simulink model "rev0BB"  (R2017b)
settings: Solver=FixedStepDiscrete  StartTime=0  StopTime=(((preLen+100+dataLenSymbols)*1+pad_first*3)*basePer)  RelTol=1e-3
values from neighbouring files (symbols this model uses):
  ack_stf_len_symbols = length(x_ACK_STF)    [rev0BB_setup.m]
  agc_delay_lag = 32    [rev0BB_setup.m]
  agc_detector_coef = ones(1,agc_detector_taps)./agc_detector_taps    [rev0BB_setup.m]
  agc_on = true    [rev0BB_startup.m]
  agc_sat_low = -agcSaturation    (= -12)    [rev0BB_setup.m]
  agc_sat_up = agcSaturation    (= 12)    [rev0BB_setup.m]
  agcDesired = 0    [rev0BB_setup.m]
  agcExpDomain = agcSaturation    (= 12)    [rev0BB_setup.m]
  agcExpResolution = 2^-5    (= 0.03125)    [rev0BB_setup.m]
  agcPwrAvgNum = 128    [rev0BB_setup.m]
  agcSaturation = 12    [rev0BB_setup.m]
  agcSettleThresh = 0.65    [rev0BB_setup.m]
  agcStep = 2^-8    (= 0.00390625)    [rev0BB_setup.m]
  atanDomain = 5    [rev0BB_setup.m]
  atanDomainTiming = 256    [rev0BB_setup.m]
  atanResolution = 2^-9    (= 0.001953125)    [rev0BB_setup.m]
  atanResolutionTiming = 2^-5    (= 0.03125)    [rev0BB_setup.m]
  averaging_num = ones(1, averaging_samples)    [rev0BB_setup.m]
  averaging_samples = 128    [rev0BB_setup.m]
  awgnSeed = abs(dBSnrRange(dBSnrInd)*1000+trial+10000000)    [plotBer.m]    (also in rev0BB_startup.m = 67)
  basePer = 1/baseFreq    (= 5e-08)    [rev0BB_setup.m]
  bitsPerSymbolHeader = log2(radixHeader)    [rev0BB_setup.m]
  bitsPerSymbolMax = log2(radixMax)    [rev0BB_setup.m]
  cal_sig_i_mult = 1.0    (= 1)    [rev0BB_startup.m]
  cal_sig_i_offset = 0.0    (= 0)    [rev0BB_startup.m]
  cal_sig_q_mult = 1.0    (= 1)    [rev0BB_startup.m]
  cal_sig_q_offset = 0.0    (= 0)    [rev0BB_startup.m]
  cefEarlyWarning = 256    [rev0BB_setup.m]
  cefLen = length(x_CEF)    [rev0BB_setup.m]
  channelFIR = zeros(1, round(maxSampleDelay)+1)    [rev0BB_startup.m]
  coarseCFOAdaptDelay = 1    [rev0BB_setup.m]
  cr_i = 0.020    (= 0.02)    [rev0BB_setup.m]
  cr_i_preamp = 2^-9    (= 0.001953125)    [rev0BB_setup.m]
  cr_int1_sat_low = -cr_integrator1_saturation    (= -0.6)    [rev0BB_setup.m]
  cr_int1_sat_up = cr_integrator1_saturation    (= 0.6)    [rev0BB_setup.m]
  cr_integrator1_decay = 1    [rev0BB_setup.m]
  cr_integrator1_saturation = 0.6    [rev0BB_setup.m]
  cr_mult_pipeline = 0    [rev0BB_setup.m]
  cr_p = 0.015    [rev0BB_setup.m]
  cr_sat2_low = -cr_saturation2    (= -0.6)    [rev0BB_setup.m]
  cr_sat2_up = cr_saturation2    (= 0.6)    [rev0BB_setup.m]
  cr_smooth_num = (1/cr_smooth_samples).*ones(1, cr_smooth_samples)    [rev0BB_setup.m]
  D_128 = [ 1,  8,  2,  4, 16, 32, 64]    [golay.m]    (also in rev0BB_setup.m)
  D_32 = [ 1,  4,  8,  2, 16]    [golay.m]    (also in rev0BB_setup.m)
  dataLenSymbols = header_len_bytes*8/bitsPerSymbolHeader + frame_len_bytes*8/bitsPerSymbol    [rev0BB_setup.m]
  default_channel = 3    [rev0BB_setup.m]
  dmm_coefs = ones(1,dmm_samples)./dmm_samples    [rev0BB_setup.m]
  dst_field_len = 8    [rev0BB_setup.m]
  expDomain = 3.3    [rev0BB_setup.m]
  expResolution = 2^-5    (= 0.03125)    [rev0BB_setup.m]
  expTol = .1    (= 0.1)    [rev0BB_setup.m]
  flush_delay = regular_pipeline*2+mult_pipeline+4    (= 4)    [rev0BB_setup.m]
  frac_lut_domain = 256    [rev0BB_setup.m]
  frac_lut_domain_cr = 64    [rev0BB_setup.m]
  frac_lut_range_max = 512    [rev0BB_setup.m]
  frac_lut_range_max_coarse_cfo = 127    [rev0BB_setup.m]
  frac_lut_range_max_cr = 127    [rev0BB_setup.m]
  frac_lut_range_min = -frac_lut_range_max    (= -512)    [rev0BB_setup.m]
  frac_lut_range_min_coarse_cfo = -frac_lut_range_max_coarse_cfo    (= -127)    [rev0BB_setup.m]
  frac_lut_range_min_cr = -frac_lut_range_max_cr    (= -127)    [rev0BB_setup.m]
  frac_lut_table_breaks = -frac_lut_domain:frac_lut_res:(frac_lut_domain-1)    [rev0BB_setup.m]
  frac_lut_table_breaks_coarse_cfo = -frac_lut_domain_coarse_cfo:frac_lut_res_coarse_cfo:(frac_lut_domain_coarse_cfo-1)    [rev0BB_setup.m]
  frac_lut_table_breaks_cr = -frac_lut_domain_cr:frac_lut_res_cr:(frac_lut_domain_cr-1)    [rev0BB_setup.m]
  frac_lut_table_data = 1./frac_lut_table_breaks    [rev0BB_setup.m]
  frac_lut_table_data_coarse_cfo = 1./frac_lut_table_breaks_coarse_cfo    [rev0BB_setup.m]
  frac_lut_table_data_cr = 1./frac_lut_table_breaks_cr    [rev0BB_setup.m]
  freeze_en_agc = true    [rev0BB_startup.m]
  freeze_en_cr_int1 = false    [rev0BB_startup.m]
  freeze_en_cr_int2 = false    [rev0BB_startup.m]
  freeze_en_cr_phase = false    [rev0BB_startup.m]
  freeze_en_tr_int1 = false    [rev0BB_startup.m]
  freeze_en_tr_int2 = false    [rev0BB_startup.m]
  freeze_en_tr_phase = false    [rev0BB_startup.m]
  freeze_on_cef_done = true    [rev0BB_startup.m]
  freeze_on_stf_done = false    [rev0BB_startup.m]
  freeze_on_valid = true    [rev0BB_startup.m]
  golay_type = 32    [rev0BB_setup.m]
  guardInt = int16(4)    [rev0BB_setup.m]
  guardTol = int16(5)    [rev0BB_setup.m]
  header_len_bytes = 8    [rev0BB_setup.m]
  lineWidth = 60    [rev0BB_setup.m]
  lmsEqDepth = 38    [rev0BB_setup.m]
  lmsStep_init = 0.006    [rev0BB_setup.m]
  lmsStep_meta = (lmsStep_final - lmsStep_init)/cefLen    [rev0BB_setup.m]
  lnDomain = 16    [rev0BB_setup.m]
  lnResolution = 2^-5    (= 0.03125)    [rev0BB_setup.m]
  local_node_id = 2    [rev0BB_startup.m]
  maxMsgSize = length(xSpectrum_PRE)+dataLenSymbols+300    [rev0BB_setup.m]
  minSTFPeaks = 3    [rev0BB_setup.m]
  mod_scheme_len_bytes = 1    [rev0BB_setup.m]
  modBPS = [1, 2, 4]    [rev0BB_setup.m]
  modKeys = [0, 1, 2]    [rev0BB_setup.m]
  mult_pipeline = 0    [rev0BB_setup.m]
  overSampleFreq = 80e6    (= 80000000)    [rev0BB_setup.m]
  overSamplePer = 1/overSampleFreq    (= 1.25e-08)    [rev0BB_setup.m]
  pad_first = 1000    [createTestVectors.m]
  post_cr_i_offset = 0    [rev0BB_startup.m]
  post_cr_q_offset = 0    [rev0BB_startup.m]
  preambleSequentialDetect = 2    [rev0BB_setup.m]
  preLen = length(x_PRE)    [rev0BB_setup.m]
  qam16_demod_scale_factor = qam16_hdl_distance/qam16_power_normalized_distance    [rev0BB_setup.m]
  rcRxFilt = [0.000303163120401141 -0.00118915940834234 -0.00187387637177 -0.00124167532697737 0.00029186889076529 0.00164526160586517 0.00182432050803312 0.000652133621739543 -0.00105668254004908 -0.00204011570659167 -0.00150058088768918 0.00026138356356816 0.0019831869994874 0.00231075800085521 0.000821993419120097 -0.00154687337975486 -0.00305430783933469 -0.00238186490079127 0.000301216962040692 0.00325307 ...(+2001 chars)    [rev0BB_setup.m]
  rcTxFilt = [0.000303163120401141 -0.00118915940834234 -0.00187387637177 -0.00124167532697737 0.00029186889076529 0.00164526160586517 0.00182432050803312 0.000652133621739543 -0.00105668254004908 -0.00204011570659167 -0.00150058088768918 0.00026138356356816 0.0019831869994874 0.00231075800085521 0.000821993419120097 -0.00154687337975486 -0.00305430783933469 -0.00238186490079127 0.000301216962040692 0.00325307 ...(+2001 chars)    [rev0BB_setup.m]
  regular_pipeline = 0    [rev0BB_setup.m]
  rx_gain = 1    [rev0BB_setup.m]
  rx_gain_i = 1    [rev0BB_setup.m]
  rx_gain_q = 1    [rev0BB_setup.m]
  rx_impare_i_offset = 0    [rev0BB_startup.m]
  rx_impare_i_scale = 1    [rev0BB_startup.m]
  rx_impare_q_offset = 0    [rev0BB_startup.m]
  rx_impare_q_scale = 1    [rev0BB_startup.m]
  rx_offset_correction_i = 0    [rev0BB_startup.m]
  rx_offset_correction_q = 0    [rev0BB_startup.m]
  sin_source_amp = 1    [rev0BB_setup.m]
  sin_source_freq = 250e6/16    (= 15625000)    [rev0BB_setup.m]
  slowPer = overSamplePer*slowSample    (= 2.5e-08)    [rev0BB_setup.m]
  std_pkt_type = 0    [rev0BB_setup.m]
  stfLen = length(x_STF)    [rev0BB_setup.m]
  testMsg = cat(1, xCTRL_PRE_adj, header, payload)    [plotBer.m]
  timing_i = 0.25    [rev0BB_setup.m]
  ... (+25 more)
undefined symbols (not defined in the file or in its folder): cr_integrator2_saturation, doppler, i, magnitude, useFadingChannel
libraries: helperLib x128, simulink x90, golayLib x34, dspsigops x32, commfilt2 x27, commdigbbndpm3 x8, hdlsllib x6, dsparch4 x4, commdigbbndam3 x4, commchan3 x2, commrflib2 x2, commcrc2 x2
(part 8 of 10)

== system rev0BB/receiver/slow_rx_baseband_outer/slow_rx_baseband_enabled/slow_rx_baseband/demod ==
  In1 : Inport
  ModMode : Inport  Port=2
  BPSK Demodulator Baseband : commdigbbndpm3/BPSK Demodulator Baseband  DecType=Hard decision  VarSource=Dialog  Variance=1  Ph=0  outDtype=uint8  derotateFactorWordLen=16  derotateFactorDataTypeStr=Inherit: Same word length as input  derotateFactorLastDataTypeStr=Inherit: Same word length as input
  Gain : Gain  Gain=qam16_demod_scale_factor
  Multiport Switch : MultiPortSwitch
  QAM16 Scale Diagram : ConstellationDiagram  Commented=on
  QPSK Demodulator Baseband : commdigbbndpm3/QPSK Demodulator Baseband  OutType=Integer  DecType=Hard decision  VarSource=Dialog  Variance=1  Dec=Gray  Ph=pi/4  outDtype1=Inherit via internal rule  outDtype2=uint8  derotateFactorWordLen=16  derotateFactorDataTypeStr=Inherit: Same word length as input  derotateFactorLastDataTypeStr=Inherit: Same word length as input
  Rectangular QAM Demodulator Baseband : commdigbbndam3/Rectangular QAM Demodulator Baseband  M=16  OutType=Integer  DecType=Hard decision  VarSource=Dialog  Variance=1  Dec=Gray  Mapping=[0:15]  PowType=Min. distance between symbols  MinDist=qam16_hdl_distance  AvgPow=1  PeakPow=1  Ph=0  outDtype1=Inherit via internal rule  outDtype2=uint8  derotateFactorWordLen=16  derotateFactorDataTypeStr=Inherit: Same word length as input  derotateFactorLastDataTypeStr=Inherit: Same word length as input  denormFactorWordLen=16  denormFactorDataTypeStr=Inherit: Same word length as input  denormFactorLastDataTypeStr=Inherit: Same word length as input  prodOutWordLen=32  prodOutOverflowMode=Wrap  prodOutRoundingMode=Floor  prodOutOvFlMode=off  prodOutOvFlModeLastStrValue=off  sumWordLen=32
  Out1 : Outport
  wires:
  BPSK Demodulator Baseband/1 -> Multiport Switch/2
  In1/1 -> QPSK Demodulator Baseband/1, Gain/1, BPSK Demodulator Baseband/1
  Multiport Switch/1 -> Out1/1
  ModMode/1 -> Multiport Switch/1
  Rectangular QAM Demodulator Baseband/1 -> Multiport Switch/4
  QPSK Demodulator Baseband/1 -> Multiport Switch/3
  Gain/1 -> QAM16 Scale Diagram/1, Rectangular QAM Demodulator Baseband/1

== system rev0BB/receiver/slow_rx_baseband_outer/slow_rx_baseband_enabled/slow_rx_baseband/freeze_logic ==
  stfDone : Inport
  cefDone : Inport  Port=2
  valid : Inport  Port=3
  freeze_on_stfDone : Inport  Port=4  OutDataTypeStr=boolean
  freeze_on_cefDone : Inport  Port=5  OutDataTypeStr=boolean
  freeze_on_valid : Inport  Port=6  OutDataTypeStr=boolean
  Logical Operator : Logic  AllPortsSameDT=off  OutDataTypeStr=boolean
  Logical Operator1 : Logic  AllPortsSameDT=off  OutDataTypeStr=boolean
  Logical Operator3 : Logic  AllPortsSameDT=off  OutDataTypeStr=boolean
  Logical Operator4 : Logic  Operator=OR  Inputs=3  AllPortsSameDT=off  OutDataTypeStr=boolean
  pipeline_delay29 : Delay  DelayLength=regular_pipeline
  pipeline_delay30 : Delay  DelayLength=regular_pipeline
  pipeline_delay32 : Delay  DelayLength=regular_pipeline
  freeze : Outport  OutDataTypeStr=boolean
  wires:
  Logical Operator4/1 -> freeze/1
  freeze_on_cefDone/1 -> pipeline_delay30/1
  freeze_on_valid/1 -> pipeline_delay32/1
  pipeline_delay30/1 -> Logical Operator1/1
  pipeline_delay29/1 -> Logical Operator/1
  valid/1 -> Logical Operator3/2
  cefDone/1 -> Logical Operator1/2
  stfDone/1 -> Logical Operator/2
  Logical Operator1/1 -> Logical Operator4/2
  pipeline_delay32/1 -> Logical Operator3/1
  freeze_on_stfDone/1 -> pipeline_delay29/1
  Logical Operator3/1 -> Logical Operator4/3
  Logical Operator/1 -> Logical Operator4/1

== system rev0BB/receiver/slow_rx_baseband_outer/slow_rx_baseband_enabled/slow_rx_baseband/header_parse_ack_decision ==
  note: min frame length of 2 symbols
  crc_decision : Inport
  crc_err : Inport  Port=2
  data : Inport  Port=3
  valid : Inport  Port=4
  local_node_id : Inport  Port=5
  Data Type Conversion{4..7} (4 alike) : DataTypeConversion  Commented=on
  Delay2 : Delay  DelayLength=1  InitialCondition=0
  Display2 : Display  Commented=on
  Logical Operator13 : Logic  Inputs=4  AllPortsSameDT=off  OutDataTypeStr=boolean
  Logical Operator14 : Logic  Operator=NOT  AllPortsSameDT=off  OutDataTypeStr=boolean
  Relational Operator : RelationalOperator  Operator===  OutDataTypeStr=boolean  RndMeth=Simplest
  Relational Operator1 : RelationalOperator  Operator===  OutDataTypeStr=boolean  RndMeth=Simplest
  Terminator{1..11} (11 alike) : Terminator
  Vector Concatenate1 : Concatenate  Commented=on  NumInputs=4
  header_parse : Stateflow chart  TreatAsAtomicUnit=on
  pipeline_delay1 : Delay  DelayLength=regular_pipeline
  pipeline_delay43 : Delay  DelayLength=regular_pipeline
  pipeline_delay44 : Delay  DelayLength=regular_pipeline
  pipeline_delay_match2 : Delay  DelayLength=regular_pipeline
  std_pkt_type : Constant  Value=std_pkt_type  OutDataTypeStr=Inherit: Inherit via back propagation  SampleTime=-1
  ack_this : Outport  SampleTime=slowPer
  ack_dst : Outport  Port=2  SampleTime=slowPer
  mod_type_valid : Outport  Port=3  SampleTime=slowPer
  mod_type : Outport  Port=4  SampleTime=slowPer
  payload_early : Outport  Port=5  SampleTime=slowPer
  payload : Outport  Port=6  SampleTime=slowPer
  wires:
  Data Type Conversion4/1 -> Vector Concatenate1/1
  Data Type Conversion5/1 -> Vector Concatenate1/2
  Data Type Conversion7/1 -> Vector Concatenate1/4
  Data Type Conversion6/1 -> Vector Concatenate1/3
  header_parse/8(type) -> pipeline_delay1/1, Terminator9/1, Data Type Conversion4/1
  crc_err/1 -> Logical Operator14/1
  header_parse/6(done_parsing) -> Terminator7/1
  valid/1 -> header_parse/2(valid)
  header_parse/4(dst_valid) -> Terminator5/1
  header_parse/5(len_valid) -> Terminator6/1
  header_parse/3(src_valid) -> Terminator4/1
  pipeline_delay_match2/1 -> ack_dst/1
  data/1 -> header_parse/1(data)
  crc_decision/1 -> Logical Operator13/1, Delay2/1
  header_parse/9(src) -> pipeline_delay_match2/1, Terminator8/1, Data Type Conversion5/1
  Logical Operator13/1 -> ack_this/1
  Delay2/1 -> header_parse/3(rst)
  Vector Concatenate1/1 -> Display2/1
  header_parse/10(dst) -> Data Type Conversion6/1, Terminator2/1, pipeline_delay44/1
  header_parse/11(len) -> Terminator1/1, Data Type Conversion7/1
  pipeline_delay44/1 -> Relational Operator/2
  header_parse/2(type_valid) -> Terminator3/1
  local_node_id/1 -> pipeline_delay43/1
  pipeline_delay43/1 -> Relational Operator/1
  Relational Operator/1 -> Logical Operator13/3
  Logical Operator14/1 -> Logical Operator13/2
  std_pkt_type/1 -> Relational Operator1/2
  Relational Operator1/1 -> Logical Operator13/4
  pipeline_delay1/1 -> Relational Operator1/1
  header_parse/1(mod_type_valid) -> mod_type_valid/1
  header_parse/7(mod_type) -> mod_type/1
  header_parse/13(payload_early) -> payload_early/1
  header_parse/12(payload) -> payload/1
  header_parse/14(net_id_valid) -> Terminator10/1
  header_parse/15(net_id) -> Terminator11/1

== system rev0BB/receiver/slow_rx_baseband_outer/slow_rx_baseband_enabled/slow_rx_baseband/mod_data_buffer ==
  data : Inport
  header : Inport  Port=2
  payload : Inport  Port=3
  last_in : Inport  Port=4
  bitsPerSymbolPayload : Inport  Port=5
  rst : Inport  Port=6
  header_parse : Stateflow chart  TreatAsAtomicUnit=on
  packed_data : Outport  SampleTime=slowPer
  valid : Outport  Port=2  SampleTime=slowPer
  last_out : Outport  Port=3  SampleTime=slowPer
  decoding : Outport  Port=4  SampleTime=slowPer
  err : Outport  Port=5  SampleTime=slowPer
  wires:
  data/1 -> header_parse/4(data)
  header/1 -> header_parse/2(header)
  header_parse/2(packed_data) -> packed_data/1
  header_parse/3(valid) -> valid/1
  header_parse/1(last_out) -> last_out/1
  payload/1 -> header_parse/5(payload)
  last_in/1 -> header_parse/1(last_in)
  bitsPerSymbolPayload/1 -> header_parse/3(bitsPerSymbolMod)
  rst/1 -> header_parse/6(rst)
  header_parse/4(decoding) -> decoding/1
  header_parse/5(err) -> err/1

== system rev0BB/receiver/slow_rx_baseband_outer/slow_rx_baseband_enabled/slow_rx_baseband/nco ==
  incr : Inport
  Data Type Conversion3 : DataTypeConversion  OutDataTypeStr=int32
  NCO : dspsigops/NCO  AccIncSrc=Input port  AccInc=100  PhaseOffsetSrc=Specify via dialog  PhaseOffset=0  AccumWL=22  HasDither=off  DitherWL=4  PNgeneratorLength=19  HasPhaseQuantizer=on  TableDepth=20  HasOutputPhaseError=off  Formula=Complex exponential  DataType=Binary point scaling  OutputWL=18  OutputFL=13  CompMethod=Table lookup (no interpolation)  SampleTime=1  SamplesPerFrame=1  OutputFrames=off
      settings: SourceProductName=DSP System Toolbox  SourceProductBaseCode=DS
  NCO HDL Optimized : dspsigops/NCO HDL Optimized  Commented=on  PhaseIncrementSource=Input port  PhaseIncrement=100  PhaseOffsetSource=Property  PhaseOffset=0  DitherSource=None  NumDitherBits=4  PhaseQuantization=on  NumQuantizerAccumulatorBits=20  LUTCompress=on  ResetAction=off  ValidInputPort=off  Waveform=Complex exponential  PhasePort=on  SimulateUsing=Code generation  AccumulatorWL=22  OutputDataType=Binary point scaling  OutputWL=18  OutputFL=13
      settings: SourceProductName=DSP System Toolbox  SourceProductBaseCode=DS
  Signal Specification : SignalSpecification  Dimensions=1
  Terminator1 : Terminator  Commented=on
  nco_phase : Scope  Commented=on
  incr_int : Outport
  complex_sin : Outport  Port=2
  wires:
  Data Type Conversion3/1 -> incr_int/1, Signal Specification/1
  Signal Specification/1 -> NCO/1
  NCO/1 -> complex_sin/1
  incr/1 -> Data Type Conversion3/1
  NCO HDL Optimized/3 -> Terminator1/1
  NCO HDL Optimized/2 -> nco_phase/1

== system rev0BB/receiver/slow_rx_baseband_outer/slow_rx_baseband_enabled/slow_rx_baseband/preamble_data_ctrl ==
  stfStart : Inport
  cefStart : Inport  Port=2
  Terminator : Terminator
  Terminator1 : Terminator
  ack_count : Scope  Commented=on
  cef_eq_fsm : Stateflow chart  TreatAsAtomicUnit=on
  data_control : Stateflow chart  TreatAsAtomicUnit=on
  dataValid : Outport
  cefSymb : Outport  Port=2
  dataLast : Outport  Port=3
  err : Outport  Port=4
  stf : Outport  Port=5
  cef : Outport  Port=6
  cefCount : Outport  Port=7
  data : Outport  Port=8
  cefEarly : Outport  Port=9
  ack : Outport  Port=10
  ack_done : Outport  Port=11
  ack_dst : Outport  Port=12
  ack_trigger : Outport  Port=13
  wires:
  cefStart/1 -> cef_eq_fsm/2(cef_start)
  stfStart/1 -> cef_eq_fsm/1(stf_start)
  cef_eq_fsm/1(data) -> data/1, data_control/1(preamble_done)
  cef_eq_fsm/3(cefSymb) -> cefSymb/1
  cef_eq_fsm/6(cefCount) -> cefCount/1
  cef_eq_fsm/7(cef_early) -> cefEarly/1
  data_control/1(valid) -> dataValid/1
  cef_eq_fsm/2(err) -> err/1
  cef_eq_fsm/4(stf) -> stf/1
  cef_eq_fsm/5(cef) -> cef/1
  data_control/2(last) -> dataLast/1
  cef_eq_fsm/8(waiting) -> Terminator/1
  cef_eq_fsm/10(ack) -> ack/1
  cef_eq_fsm/9(ack_done) -> ack_done/1
  cef_eq_fsm/11(ack_dst) -> ack_dst/1
  cef_eq_fsm/12(ack_count) -> Terminator1/1, ack_count/1
  cef_eq_fsm/13(ack_trigger) -> ack_trigger/1

== system rev0BB/receiver/fast_rx_baseband/Timing Recovery/nda_4x_time_err_enable/phase_est/timing_rec_sym_rate_enb ==
  delay3 : Inport
  delay2 : Inport  Port=2
  delay1 : Inport  Port=3
  delay0 : Inport  Port=4
  Data Type Conversion1 : DataTypeConversion  OutDataTypeStr=single
  Data Type Conversion2 : DataTypeConversion  OutDataTypeStr=single
  Discrete FIR Filter : DiscreteFir  Commented=on  FilterStructure=Direct form transposed  Coefficients=averaging_num  OutDataTypeStr=Inherit: Same as input
  Discrete FIR Filter1 : DiscreteFir  Commented=on  FilterStructure=Direct form transposed  Coefficients=averaging_num  OutDataTypeStr=Inherit: Same as input
  Gain1 : Gain  Gain=1/4  OutDataTypeStr=Inherit: Same as input
  Gain2 : Gain  Gain=1/4  OutDataTypeStr=Inherit: Same as input
  Sub : Sum  Inputs=+-  OutDataTypeStr=Inherit: Same as first input
  Sub1 : Sum  Inputs=-+  OutDataTypeStr=Inherit: Same as first input
  Trigonometric Function : Trigonometry  Operator=atan2
  atan2 : Subsystem  Commented=on  AncestorBlock=helperLib/atan2
  average_filter : Subsystem  AncestorBlock=helperLib/average_filter  mask{pipe=regular_pipeline, samples=averaging_samples, gain=1}
      mask prompts: pipe "Pipeline Delay"; samples "Samples to Average Over"; gain "Gain to Multiply Each Sample By"
  average_filter1 : Subsystem  AncestorBlock=helperLib/average_filter  mask{pipe=regular_pipeline, samples=averaging_samples, gain=1}
      mask prompts: pipe "Pipeline Delay"; samples "Samples to Average Over"; gain "Gain to Multiply Each Sample By"
  pipeline_delay{,1..4,6..7} (7 alike) : Delay  DelayLength=regular_pipeline
  pipelined_gain : helperLib/pipelined_gain  g=-1/(2*pi)  d=wide_mult_pipeline
  err : Outport
  wires:
  pipeline_delay2/1 -> err/1
  delay3/1 -> Sub/1
  delay0/1 -> Sub1/2
  Sub1/1 -> pipeline_delay1/1
  delay1/1 -> Sub/2
  delay2/1 -> Sub1/1
  Sub/1 -> pipeline_delay/1
  Trigonometric Function/1 -> pipelined_gain/1
  pipelined_gain/1 -> pipeline_delay2/1
  Data Type Conversion1/1 -> pipeline_delay6/1
  Gain2/1 -> Data Type Conversion2/1
  pipeline_delay6/1 -> Trigonometric Function/1
  pipeline_delay7/1 -> Trigonometric Function/2
  average_filter1/1(Out1) -> pipeline_delay4/1
  average_filter/1(Out1) -> pipeline_delay3/1
  pipeline_delay/1 -> average_filter/1(In1)
  pipeline_delay1/1 -> average_filter1/1(In1)
  pipeline_delay4/1 -> Gain2/1
  pipeline_delay3/1 -> Gain1/1
  Gain1/1 -> Data Type Conversion1/1
  Data Type Conversion2/1 -> pipeline_delay7/1

== system rev0BB/receiver/slow_rx_baseband_outer/slow_rx_baseband_enabled/slow_rx_baseband/CoarseCFO_est/atan ==
  note: 5 delays
  note: Special case for undefined ouput of atan2.
      | To produce an unbiased ouput, this should be 0.
  imag_y : Inport
  real_x : Inport  Port=2
  Compare To Constant2 : simulink/Logic and Bit Operations/Compare To Constant  relop=>=  const=0  OutDataTypeStr=boolean
  Compare To Constant3 : simulink/Logic and Bit Operations/Compare To Constant  relop===  const=0  OutDataTypeStr=boolean
  Compare To Constant4 : simulink/Logic and Bit Operations/Compare To Constant  relop===  const=0  OutDataTypeStr=boolean
  Constant2 : Constant  Value=0  OutDataTypeStr=Inherit: Inherit via back propagation  SampleTime=-1
  Constant3 : Constant  Value=-pi/2  OutDataTypeStr=Inherit: Inherit via back propagation  SampleTime=-1
  Constant4 : Constant  Value=pi/2  OutDataTypeStr=Inherit: Inherit via back propagation  SampleTime=-1
  Logical Operator : Logic  AllPortsSameDT=off  OutDataTypeStr=boolean
  Logical Operator1 : Logic  AllPortsSameDT=off  OutDataTypeStr=boolean
  Switch3 : Switch  Criteria=u2 ~= 0  OutDataTypeStr=Inherit: Inherit via back propagation
  Switch4 : Switch  Criteria=u2 ~= 0  OutDataTypeStr=Inherit: Inherit via back propagation
  Switch5 : Switch  Criteria=u2 ~= 0  OutDataTypeStr=Inherit: Inherit via back propagation
  bound_atan : Subsystem  AncestorBlock=helperLib/bound_atan
  inv : Subsystem
  mult_delay_match : Delay  DelayLength=cr_mult_pipeline*2+regular_pipeline*2
  pipeline_delay{,1..3} (4 alike) : Delay  DelayLength=regular_pipeline
  pipeline_delay_match2 : Delay  DelayLength=cr_mult_pipeline*5+regular_pipeline*7
  pipeline_delay_match3 : Delay  DelayLength=cr_mult_pipeline*5+regular_pipeline*7
  pipeline_delay_match4 : Delay  DelayLength=cr_mult_pipeline*5+regular_pipeline*7
  pipelined_mult : helperLib/pipelined_mult  d=cr_mult_pipeline
  Out1 : Outport
  wires:
  pipeline_delay1/1 -> bound_atan/1(In1)
  imag_y/1 -> Compare To Constant4/1, Compare To Constant2/1, mult_delay_match/1
  mult_delay_match/1 -> pipeline_delay2/1
  bound_atan/1(Out1) -> pipeline_delay/1
  pipelined_mult/1 -> pipeline_delay1/1
  pipeline_delay2/1 -> pipelined_mult/1
  pipeline_delay3/1 -> pipelined_mult/2
  Compare To Constant4/1 -> Logical Operator/1
  Logical Operator/1 -> pipeline_delay_match2/1
  pipeline_delay_match2/1 -> Switch3/2
  real_x/1 -> inv/1(In), Compare To Constant3/1
  inv/1(Out) -> pipeline_delay3/1
  Switch4/1 -> Switch5/3
  Constant3/1 -> Switch4/1
  Constant4/1 -> Switch5/1
  Switch5/1 -> Switch3/3
  Constant2/1 -> Switch3/1
  Compare To Constant3/1 -> Logical Operator1/2, pipeline_delay_match4/1, Logical Operator/2
  Logical Operator1/1 -> pipeline_delay_match3/1
  pipeline_delay_match3/1 -> Switch5/2
  pipeline_delay_match4/1 -> Switch4/2
  Compare To Constant2/1 -> Logical Operator1/1
  pipeline_delay/1 -> Switch4/3
  Switch3/1 -> Out1/1

== system rev0BB/receiver/slow_rx_baseband_outer/slow_rx_baseband_enabled/slow_rx_baseband/CoarseCFO_est/complex_mult_pipelined1 ==
  In1 : Inport
  In2 : Inport  Port=2
  Add1 : Sum  OutDataTypeStr=Inherit: Same as first input
  Add2 : Sum  OutDataTypeStr=Inherit: Same as first input
  Complex to Real-Imag3 : ComplexToRealImag
  Complex to Real-Imag4 : ComplexToRealImag
  Real-Imag to Complex2 : RealImagToComplex
  mult_delay_match3 : Delay  DelayLength=cr_mult_pipeline
  mult_delay_match4 : Delay  DelayLength=cr_mult_pipeline
  mult_delay_match5 : Delay  DelayLength=cr_mult_pipeline
  pipeline_delay{1..3,6} (4 alike) : Delay  DelayLength=regular_pipeline
  pipelined_gain : helperLib/pipelined_gain  g=-1  d=cr_mult_pipeline
  pipelined_mult{,1..3} (4 alike) : helperLib/pipelined_mult  d=cr_mult_pipeline
  Out1 : Outport
  wires:
  pipelined_gain/1 -> Add1/2
  pipelined_mult3/1 -> mult_delay_match5/1
  pipelined_mult2/1 -> mult_delay_match4/1
  pipelined_mult1/1 -> pipelined_gain/1
  pipelined_mult/1 -> mult_delay_match3/1
  Complex to Real-Imag4/1 -> pipelined_mult/2, pipelined_mult3/2
  Complex to Real-Imag3/2 -> pipelined_mult1/1, pipelined_mult3/1
  Complex to Real-Imag4/2 -> pipelined_mult2/2, pipelined_mult1/2
  Complex to Real-Imag3/1 -> pipelined_mult2/1, pipelined_mult/1
  pipeline_delay3/1 -> Complex to Real-Imag4/1
  pipeline_delay2/1 -> Complex to Real-Imag3/1
  Add2/1 -> pipeline_delay6/1
  Add1/1 -> pipeline_delay1/1
  In1/1 -> pipeline_delay2/1
  mult_delay_match5/1 -> Add2/2
  pipeline_delay1/1 -> Real-Imag to Complex2/1
  In2/1 -> pipeline_delay3/1
  pipeline_delay6/1 -> Real-Imag to Complex2/2
  Real-Imag to Complex2/1 -> Out1/1
  mult_delay_match3/1 -> Add1/1
  mult_delay_match4/1 -> Add2/1

== system rev0BB/receiver/slow_rx_baseband_outer/slow_rx_baseband_enabled/slow_rx_baseband/EQ/lms ==
  in : Inport
  expected : Inport  Port=2
  reset : Inport  Port=3
  adapt : Inport  Port=4
  step : Inport  Port=5
  Data Type Conversion : DataTypeConversion  OutDataTypeStr=single
  Data Type Conversion1 : DataTypeConversion  OutDataTypeStr=single
  Data Type Conversion2 : DataTypeConversion  OutDataTypeStr=single
  Delay3 : Delay  DelayLength=lmsEqDepth/2-1  InitialCondition=0
  Discrete FIR Filter : DiscreteFir  CoefSource=Input port  FilterStructure=Direct form transposed  ProductDataTypeStr=fixdt(1,17,12)  AccumDataTypeStr=fixdt(1,17,12)  OutDataTypeStr=fixdt(1,25,19)
      settings: InputPortMap=u0,u1
  Display : Display  Commented=on
  Product : Product  OutDataTypeStr=Inherit: Same as first input
  Product1 : Product  OutDataTypeStr=Inherit: Same as first input
  Sum : Sum  Inputs=|+-  OutDataTypeStr=Inherit: Same as first input
  Sum1 : Sum  Inputs=|++  OutDataTypeStr=Inherit: Same as first input
  Switch : Switch  Criteria=u2 > Threshold
  Tapped Delay : simulink/Discrete/Tapped Delay  vinit=0.0  samptime=-1  NumDelays=lmsEqDepth-1  DelayOrder=Newest  includeCurrent=off
  Unit Delay Resettable : simulink_need_slupdate/Unit Delay Resettable  vinit=complex(cat(1,zeros(lmsEqDepth/2-1,1), [1], zeros(lmsEqDepth/2,1)))  tsamp=-1
      settings: SourceProductName=Simulink  SourceProductBaseCode=SL
  Vector Concatenate : Concatenate
  complex_conj : helperLib/complex_conj
  pipeline_delay{1,3..6} (5 alike) : Delay  DelayLength=regular_pipeline
  out : Outport
  err : Outport  Port=2
  weights : Outport  Port=3
  wires:
  Tapped Delay/1 -> Vector Concatenate/2
  Data Type Conversion2/1 -> pipeline_delay6/1
  complex_conj/1 -> Tapped Delay/1, Vector Concatenate/1
  Sum1/1 -> Switch/1
  Data Type Conversion1/1 -> pipeline_delay1/1
  Data Type Conversion/1 -> Delay3/1
  step/1 -> pipeline_delay3/1
  Delay3/1 -> pipeline_delay4/1
  adapt/1 -> Switch/2
  pipeline_delay1/1 -> complex_conj/1, Discrete FIR Filter/1
  Unit Delay Resettable/1 -> Sum1/1, Display/1, Switch/3, Discrete FIR Filter/2, weights/1
  Switch/1 -> Unit Delay Resettable/1
  reset/1 -> Unit Delay Resettable/2
  expected/1 -> Data Type Conversion/1
  in/1 -> Data Type Conversion1/1
  pipeline_delay5/1 -> err/1
  pipeline_delay6/1 -> out/1
  Sum/1 -> Product/1, pipeline_delay5/1
  pipeline_delay3/1 -> Product/2
  Product/1 -> Product1/1
  Vector Concatenate/1 -> Product1/2
  pipeline_delay4/1 -> Sum/1
  Discrete FIR Filter/1 -> Sum/2, Data Type Conversion2/1
  Product1/1 -> Sum1/2

== system rev0BB/receiver/slow_rx_baseband_outer/slow_rx_baseband_enabled/slow_rx_baseband/FineCarrierRecovery/Est_Phase ==
  In1 : Inport
  ModMode : Inport  Port=2
  Complex to Real-Imag : ComplexToRealImag
  Complex to Real-Imag1 : ComplexToRealImag
  Data Type Conversion : DataTypeConversion  OutDataTypeStr=single
  Gain : Gain  Gain=-1  OutDataTypeStr=Inherit: Same as input
  Real-Imag to Complex1 : RealImagToComplex
  Trigonometric Function : Trigonometry  Operator=atan2
  atan2 : Subsystem  Commented=on  AncestorBlock=helperLib/atan2
  complex_mult_pipelined1 : Subsystem  AncestorBlock=helperLib/complex_mult_pipelined
  find_nearest : Subsystem
  mult_delay5 : Delay  DelayLength=cr_mult_pipeline
  mult_delay_match : Delay  DelayLength=cr_mult_pipeline
  mult_delay_match2 : Delay  DelayLength=cr_mult_pipeline
  pipeline_delay2 : Delay  DelayLength=regular_pipeline
  phase_offset : Outport
  wires:
  mult_delay_match2/1 -> complex_mult_pipelined1/1(In1)
  find_nearest/1(Out1) -> mult_delay_match2/1
  Data Type Conversion/1 -> Complex to Real-Imag/1, find_nearest/1(In1)
  Trigonometric Function/1 -> pipeline_delay2/1
  Complex to Real-Imag1/2 -> Trigonometric Function/1
  Complex to Real-Imag1/1 -> Trigonometric Function/2
  pipeline_delay2/1 -> phase_offset/1
  Gain/1 -> Real-Imag to Complex1/2
  mult_delay_match/1 -> Real-Imag to Complex1/1
  Real-Imag to Complex1/1 -> complex_mult_pipelined1/2(In2)
  Complex to Real-Imag/2 -> mult_delay5/1
  Complex to Real-Imag/1 -> mult_delay_match/1
  In1/1 -> Data Type Conversion/1
  mult_delay5/1 -> Gain/1
  complex_mult_pipelined1/1(Out1) -> Complex to Real-Imag1/1
  ModMode/1 -> find_nearest/2(ModMode)

== system rev0BB/receiver/slow_rx_baseband_outer/slow_rx_baseband_enabled/slow_rx_baseband/FineCarrierRecovery/PostCR_IQ_Offset_Correct ==
  In : Inport
  post_cr_i_offset : Inport  Port=2
  post_cr_q_offset : Inport  Port=3
  Add : Sum  OutDataTypeStr=Inherit: Same as first input
  Add1 : Sum  OutDataTypeStr=Inherit: Same as first input
  Complex to Real-Imag1 : ComplexToRealImag
  Real-Imag to Complex1 : RealImagToComplex
  pipeline_delay : Delay  DelayLength=regular_pipeline
  pipeline_delay1 : Delay  DelayLength=regular_pipeline
  Out : Outport
  wires:
  Real-Imag to Complex1/1 -> Out/1
  Add/1 -> pipeline_delay/1
  Complex to Real-Imag1/2 -> Add1/1
  Complex to Real-Imag1/1 -> Add/1
  Add1/1 -> pipeline_delay1/1
  In/1 -> Complex to Real-Imag1/1
  post_cr_q_offset/1 -> Add1/2
  post_cr_i_offset/1 -> Add/2
  pipeline_delay/1 -> Real-Imag to Complex1/1
  pipeline_delay1/1 -> Real-Imag to Complex1/2

== system rev0BB/receiver/slow_rx_baseband_outer/slow_rx_baseband_enabled/slow_rx_baseband/FineCarrierRecovery/complex_mult_pipelined ==
  In1 : Inport
  In2 : Inport  Port=2
  Add1 : Sum  OutDataTypeStr=Inherit: Same as first input
  Add2 : Sum  OutDataTypeStr=Inherit: Same as first input
  Complex to Real-Imag3 : ComplexToRealImag
  Complex to Real-Imag4 : ComplexToRealImag
  Real-Imag to Complex2 : RealImagToComplex
  mult_delay_match3 : Delay  DelayLength=cr_mult_pipeline
  mult_delay_match4 : Delay  DelayLength=cr_mult_pipeline
  mult_delay_match5 : Delay  DelayLength=cr_mult_pipeline
  pipeline_delay{1..3,6} (4 alike) : Delay  DelayLength=regular_pipeline
  pipelined_gain : helperLib/pipelined_gain  g=-1  d=cr_mult_pipeline
  pipelined_mult{,1..3} (4 alike) : helperLib/pipelined_mult  d=cr_mult_pipeline
  Out1 : Outport
  wires:
  pipelined_gain/1 -> Add1/2
  pipelined_mult3/1 -> mult_delay_match5/1
  pipelined_mult2/1 -> mult_delay_match4/1
  pipelined_mult1/1 -> pipelined_gain/1
  pipelined_mult/1 -> mult_delay_match3/1
  Complex to Real-Imag4/1 -> pipelined_mult/2, pipelined_mult3/2
  Complex to Real-Imag3/2 -> pipelined_mult1/1, pipelined_mult3/1
  Complex to Real-Imag4/2 -> pipelined_mult2/2, pipelined_mult1/2
  Complex to Real-Imag3/1 -> pipelined_mult2/1, pipelined_mult/1
  pipeline_delay3/1 -> Complex to Real-Imag4/1
  pipeline_delay2/1 -> Complex to Real-Imag3/1
  Add2/1 -> pipeline_delay6/1
  Add1/1 -> pipeline_delay1/1
  In1/1 -> pipeline_delay2/1
  mult_delay_match5/1 -> Add2/2
  pipeline_delay1/1 -> Real-Imag to Complex2/1
  In2/1 -> pipeline_delay3/1
  pipeline_delay6/1 -> Real-Imag to Complex2/2
  Real-Imag to Complex2/1 -> Out1/1
  mult_delay_match3/1 -> Add1/1
  mult_delay_match4/1 -> Add2/1

== system rev0BB/receiver/slow_rx_baseband_outer/slow_rx_baseband_enabled/slow_rx_baseband/FineCarrierRecovery/overflow_protect ==
  note: Synthesizer
  note: This fixes overflow problem with LUT.  This keeps the
      | signal from -pi to pi plus some hystoresis if the LUT's
      | domain is slightly larger than -pi to pi
  In1 : Inport
  Compare To Constant2 : simulink/Logic and Bit Operations/Compare To Constant  relop=>=  const=expDomain-expTol  OutDataTypeStr=boolean
  Compare To Constant3 : simulink/Logic and Bit Operations/Compare To Constant  relop=<=  const=-expDomain+expTol  OutDataTypeStr=boolean
  Constant1 : Constant  Value=2*pi  OutDataTypeStr=Inherit: Inherit via back propagation  SampleTime=-1
  Constant2 : Constant  Value=0  OutDataTypeStr=Inherit: Inherit via back propagation  SampleTime=-1
  Sum4 : Sum  Inputs=|+-  OutDataTypeStr=Inherit: Same as first input
  Sum5 : Sum  Inputs=|++  OutDataTypeStr=Inherit: Same as first input
  Switch : Switch  Criteria=u2 ~= 0  OutDataTypeStr=Inherit: Inherit via back propagation
  Switch1 : Switch  Criteria=u2 ~= 0  OutDataTypeStr=Inherit: Inherit via back propagation
  Out1 : Outport
  wires:
  Sum4/1 -> Out1/1
  Compare To Constant3/1 -> Switch/2
  Compare To Constant2/1 -> Switch1/2
  Constant1/1 -> Switch/1, Switch1/1
  Constant2/1 -> Switch1/3, Switch/3
  Switch/1 -> Sum5/2
  Sum5/1 -> Sum4/1
  Switch1/1 -> Sum4/2
  In1/1 -> Sum5/1, Compare To Constant3/1, Compare To Constant2/1

== system rev0BB/receiver/slow_rx_baseband_outer/slow_rx_baseband_enabled/slow_rx_baseband/FineCarrierRecovery/scale_and_loop ==
  phase_offset : Inport
  cr_i_preamp : Inport  Port=2
  cr_p : Inport  Port=3
  cr_i : Inport  Port=4
  cr_integrator1_decay : Inport  Port=5
  cr_int1_sat_up : Inport  Port=6
  cr_int1_sat_low : Inport  Port=7
  cr_sat2_up : Inport  Port=8
  cr_sat2_low : Inport  Port=9
  cr_int1_freeze : Inport  Port=10
  reset : Inport  Port=11
  Loop Filter : Subsystem
  pipeline_delay8 : Delay  DelayLength=regular_pipeline
  correction : Outport
  wires:
  Loop Filter/1(Out) -> pipeline_delay8/1
  phase_offset/1 -> Loop Filter/1(PhaseOffset)
  pipeline_delay8/1 -> correction/1
  cr_i_preamp/1 -> Loop Filter/2(cr_i_preamp)
  cr_p/1 -> Loop Filter/3(cr_p)
  cr_i/1 -> Loop Filter/4(cr_i)
  cr_integrator1_decay/1 -> Loop Filter/5(cr_integrator1_decay)
  cr_sat2_low/1 -> Loop Filter/9(cr_sat2_low)
  cr_sat2_up/1 -> Loop Filter/8(cr_sat2_up)
  cr_int1_sat_low/1 -> Loop Filter/7(cr_int1_sat_low)
  cr_int1_sat_up/1 -> Loop Filter/6(cr_int1_sat_up)
  cr_int1_freeze/1 -> Loop Filter/10(int1_freeze)
  reset/1 -> Loop Filter/11(reset)

== system rev0BB/receiver/slow_rx_baseband_outer/slow_rx_baseband_enabled/slow_rx_baseband/FineCarrierRecovery/shift180 ==
  note: Todo: propogate this conversion back
  In1 : Inport
  shift180 : Inport  Port=2
  Constant8 : Constant  Value=0  OutDataTypeStr=Inherit: Inherit via back propagation  SampleTime=-1
  Constant9 : Constant  Value=pi  OutDataTypeStr=Inherit: Inherit via back propagation  SampleTime=-1
  Sum6 : Sum  Inputs=|++  OutDataTypeStr=Inherit: Same as first input
  Switch6 : Switch  Criteria=u2 ~= 0  OutDataTypeStr=Inherit: Inherit via back propagation
  pipeline_delay_match1 : Delay  DelayLength=regular_pipeline
  Out1 : Outport
  wires:
  In1/1 -> Sum6/1
  shift180/1 -> pipeline_delay_match1/1
  Constant9/1 -> Switch6/1
  Constant8/1 -> Switch6/3
  Sum6/1 -> Out1/1
  Switch6/1 -> Sum6/2
  pipeline_delay_match1/1 -> Switch6/2

== system rev0BB/receiver/fast_rx_baseband/Timing Recovery/nda_4x_time_err_enable/phase_est/timing_rec_sym_rate_enb/atan2 ==
  note: Special case for undefined ouput of atan2.
      | To produce an unbiased ouput, this should be 0.
  note: 4 delays
  note: 9 delays
  imag_y : Inport
  real_x : Inport  Port=2
  Add : Sum  OutDataTypeStr=Inherit: Same as first input
  Compare To Constant1 : simulink/Logic and Bit Operations/Compare To Constant  relop=>  const=0  OutDataTypeStr=boolean
  Compare To Constant2 : simulink/Logic and Bit Operations/Compare To Constant  relop=>=  const=0  OutDataTypeStr=boolean
  Compare To Constant3 : simulink/Logic and Bit Operations/Compare To Constant  relop===  const=0  OutDataTypeStr=boolean
  Compare To Constant4 : simulink/Logic and Bit Operations/Compare To Constant  relop===  const=0  OutDataTypeStr=boolean
  Constant : Constant  Value=pi  OutDataTypeStr=Inherit: Inherit via back propagation  SampleTime=-1
  Constant1 : Constant  Value=0  OutDataTypeStr=Inherit: Inherit via back propagation  SampleTime=-1
  Constant2 : Constant  Value=-pi/2  OutDataTypeStr=Inherit: Inherit via back propagation  SampleTime=-1
  Constant3 : Constant  Value=pi/2  OutDataTypeStr=Inherit: Inherit via back propagation  SampleTime=-1
  Logical Operator : Logic  AllPortsSameDT=off  OutDataTypeStr=boolean
  Logical Operator1 : Logic  AllPortsSameDT=off  OutDataTypeStr=boolean
  Sub : Sum  Inputs=-+  OutDataTypeStr=Inherit: Same as first input
  Switch{1..4,8} (5 alike) : Switch  Criteria=u2 ~= 0  OutDataTypeStr=Inherit: Inherit via back propagation
  bound_atan : Subsystem  AncestorBlock=helperLib/bound_atan
  inv : Subsystem
  mult_delay_match : Delay  DelayLength=wide_mult_pipeline+regular_pipeline*4
  mult_delay_match1 : Delay  DelayLength=regular_pipeline
  pipeline_delay{,1..3} (4 alike) : Delay  DelayLength=regular_pipeline
  pipeline_delay_match{,1..4} (5 alike) : Delay  DelayLength=regular_pipeline*12+wide_mult_pipeline*3
  pipelined_mult : helperLib/pipelined_mult  d=wide_mult_pipeline
  Out1 : Outport
  wires:
  pipeline_delay_match/1 -> Switch1/2
  pipeline_delay_match1/1 -> Switch8/2
  Sub/1 -> Switch1/3
  Constant/1 -> Sub/1, Add/2
  Add/1 -> Switch1/1
  Switch1/1 -> Switch8/3
  Compare To Constant2/1 -> Logical Operator1/1, pipeline_delay_match/1
  Compare To Constant1/1 -> pipeline_delay_match1/1
  pipeline_delay/1 -> Sub/2, Switch8/1, Add/1
  imag_y/1 -> Compare To Constant4/1, pipeline_delay1/1, Compare To Constant2/1
  real_x/1 -> pipeline_delay2/1, Compare To Constant3/1, Compare To Constant1/1
  pipeline_delay1/1 -> mult_delay_match/1
  pipeline_delay2/1 -> inv/1(In)
  bound_atan/1(Out1) -> pipeline_delay/1
  pipelined_mult/1 -> bound_atan/1(In1)
  Compare To Constant3/1 -> Logical Operator/2, Logical Operator1/2, pipeline_delay_match3/1
  Switch8/1 -> Switch3/3
  Compare To Constant4/1 -> Logical Operator/1
  Logical Operator/1 -> pipeline_delay_match2/1
  Switch3/1 -> Switch4/3
  Constant2/1 -> Switch3/1
  Logical Operator1/1 -> pipeline_delay_match4/1
  Constant3/1 -> Switch4/1
  Switch4/1 -> Switch2/3
  Constant1/1 -> Switch2/1
  Switch2/1 -> Out1/1
  pipeline_delay_match2/1 -> Switch2/2
  pipeline_delay_match3/1 -> Switch3/2
  pipeline_delay_match4/1 -> Switch4/2
  pipeline_delay3/1 -> pipelined_mult/2
  mult_delay_match1/1 -> pipelined_mult/1
  mult_delay_match/1 -> mult_delay_match1/1
  inv/1(Out) -> pipeline_delay3/1

== system rev0BB/receiver/fast_rx_baseband/Timing Recovery/nda_4x_time_err_enable/phase_est/timing_rec_sym_rate_enb/average_filter ==
  note: Clever Arch of an Averaging Filter I saw in A Split MAC Approach for SDR Platforms by Paolo Di Francesco, S´eamas McGettrick, Uchenna K. Anyanwu, James C. O’Sullivan,
      | Allen B. MacKenzie, and Luiz A. DaSilva.  This requires a shift register, 1 mult, and 2 adds (3 if you count the negation).  Downside is unpipelined loopback (standard IIR problem)
  In1 : Inport
  Data Type Conversion : DataTypeConversion
  Delay : Delay  DelayLength=samples  InitialCondition=0
  Delay1 : Delay  DelayLength=1  InitialCondition=0
  Gain : Gain  Gain=gain  OutDataTypeStr=Inherit: Same as input
  Sum : Sum  Inputs=|++  OutDataTypeStr=Inherit: Same as first input
  Sum1 : Sum  Inputs=|+-  OutDataTypeStr=Inherit: Same as first input
  pipeline_delay : Delay  DelayLength=pipe
  Out1 : Outport
  wires:
  Data Type Conversion/1 -> Sum/1
  pipeline_delay/1 -> Data Type Conversion/1, Delay/1
  Gain/1 -> pipeline_delay/1
  Delay1/1 -> Sum/2
  Sum1/1 -> Delay1/1, Out1/1
  Delay/1 -> Sum1/2
  In1/1 -> Gain/1
  Sum/1 -> Sum1/1

== system rev0BB/receiver/fast_rx_baseband/Timing Recovery/nda_4x_time_err_enable/phase_est/timing_rec_sym_rate_enb/average_filter1 ==
  note: Clever Arch of an Averaging Filter I saw in A Split MAC Approach for SDR Platforms by Paolo Di Francesco, S´eamas McGettrick, Uchenna K. Anyanwu, James C. O’Sullivan,
      | Allen B. MacKenzie, and Luiz A. DaSilva.  This requires a shift register, 1 mult, and 2 adds (3 if you count the negation).  Downside is unpipelined loopback (standard IIR problem)
  In1 : Inport
  Data Type Conversion : DataTypeConversion
  Delay : Delay  DelayLength=samples  InitialCondition=0
  Delay1 : Delay  DelayLength=1  InitialCondition=0
  Gain : Gain  Gain=gain  OutDataTypeStr=Inherit: Same as input
  Sum : Sum  Inputs=|++  OutDataTypeStr=Inherit: Same as first input
  Sum1 : Sum  Inputs=|+-  OutDataTypeStr=Inherit: Same as first input
  pipeline_delay : Delay  DelayLength=pipe
  Out1 : Outport
  wires:
  Data Type Conversion/1 -> Sum/1
  pipeline_delay/1 -> Data Type Conversion/1, Delay/1
  Gain/1 -> pipeline_delay/1
  Delay1/1 -> Sum/2
  Sum1/1 -> Delay1/1, Out1/1
  Delay/1 -> Sum1/2
  In1/1 -> Gain/1
  Sum/1 -> Sum1/1

== system rev0BB/receiver/slow_rx_baseband_outer/slow_rx_baseband_enabled/slow_rx_baseband/CoarseCFO_est/atan/bound_atan ==
  note: Bound Protection
  In1 : Inport
  Compare To Constant1 : simulink/Logic and Bit Operations/Compare To Constant  relop=>=  const=atanDomain  OutDataTypeStr=boolean
  Compare To Constant4 : simulink/Logic and Bit Operations/Compare To Constant  relop=<=  const=-atanDomain  OutDataTypeStr=boolean
  Constant11 : Constant  Value=0  OutDataTypeStr=Inherit: Inherit via back propagation  SampleTime=-1
  Constant3 : Constant  Value=pi/2  OutDataTypeStr=Inherit: Inherit via back propagation  SampleTime=-1
  Constant4 : Constant  Value=-pi/2  OutDataTypeStr=Inherit: Inherit via back propagation  SampleTime=-1
  Data Type Duplicate : DataTypeDuplicate
  Data Type Duplicate1 : DataTypeDuplicate
  Data Type Duplicate2 : DataTypeDuplicate
  Data Type Conversion : DataTypeConversion  OutDataTypeStr=single
  Logical Operator : Logic  Operator=OR  AllPortsSameDT=off  OutDataTypeStr=boolean
  Switch2 : Switch  Criteria=u2 ~= 0  OutDataTypeStr=Inherit: Inherit via back propagation
  Switch3 : Switch  Criteria=u2 ~= 0  OutDataTypeStr=Inherit: Inherit via back propagation
  Switch8 : Switch  Criteria=u2 ~= 0  OutDataTypeStr=Inherit: Inherit via back propagation
  atan Lookup Table : Lookup_n-D  NumberOfTableDimensions=1  BreakpointsForDimension1=[-atanDomain:atanResolution:atanDomain]  IndexSearchMethod=Evenly spaced points  Table=atan([-atanDomain:atanResolution:atanDomain])  InterpMethod=Flat  DiagnosticForOutOfRangeInput=Error  RemoveProtectionInput=on  InternalRulePriority=Speed  OutDataTypeStr=Inherit: Inherit via back propagation  RndMeth=Simplest  InputSameDT=on
  mult_delay : Delay  DelayLength=cr_mult_pipeline
  mult_delay_match : Delay  DelayLength=cr_mult_pipeline
  mult_delay_match1 : Delay  DelayLength=cr_mult_pipeline
  pipeline_delay1 : Delay  DelayLength=regular_pipeline*2
  pipeline_delay2 : Delay  DelayLength=regular_pipeline
  pipeline_delay_match : Delay  DelayLength=regular_pipeline*3
  pipeline_delay_match1 : Delay  DelayLength=regular_pipeline*3
  Out1 : Outport
  wires:
  pipeline_delay2/1 -> Data Type Duplicate2/1, Switch2/3
  mult_delay/1 -> atan Lookup Table/1
  pipeline_delay1/1 -> mult_delay/1
  mult_delay_match1/1 -> Switch3/2
  mult_delay_match/1 -> Switch2/2
  pipeline_delay_match1/1 -> mult_delay_match1/1
  pipeline_delay_match/1 -> mult_delay_match/1
  atan Lookup Table/1 -> Data Type Duplicate/2, pipeline_delay2/1
  Switch8/1 -> Data Type Conversion/1
  Constant11/1 -> Switch8/1
  Logical Operator/1 -> Switch8/2
  In1/1 -> Data Type Duplicate/1, Compare To Constant4/1, Compare To Constant1/1, Switch8/3
  Switch3/1 -> Data Type Duplicate2/2, Data Type Duplicate1/2, Out1/1
  Constant4/1 -> Switch3/1
  Switch2/1 -> Data Type Duplicate1/1, Switch3/3
  Constant3/1 -> Switch2/1
  Compare To Constant4/1 -> pipeline_delay_match1/1, Logical Operator/2
  Compare To Constant1/1 -> pipeline_delay_match/1, Logical Operator/1
  Data Type Conversion/1 -> pipeline_delay1/1

== system rev0BB/receiver/slow_rx_baseband_outer/slow_rx_baseband_enabled/slow_rx_baseband/CoarseCFO_est/atan/inv ==
  note: Bound Protection
  In : Inport
  Compare To Constant1 : simulink/Logic and Bit Operations/Compare To Constant  relop=>=  const=frac_lut_domain_cr-1  OutDataTypeStr=boolean
  Compare To Constant4 : simulink/Logic and Bit Operations/Compare To Constant  relop=<=  const=-frac_lut_domain_cr  OutDataTypeStr=boolean
  Constant11 : Constant  Value=0  OutDataTypeStr=Inherit: Inherit via back propagation  SampleTime=-1
  Constant3 : Constant  Value=frac_lut_range_max_coarse_cfo  OutDataTypeStr=Inherit: Inherit via back propagation  SampleTime=-1
  Constant4 : Constant  Value=frac_lut_range_min_coarse_cfo  OutDataTypeStr=Inherit: Inherit via back propagation  SampleTime=-1
  Data Type Duplicate : DataTypeDuplicate
  Data Type Duplicate1 : DataTypeDuplicate
  Data Type Duplicate2 : DataTypeDuplicate
  Data Type Conversion : DataTypeConversion  OutDataTypeStr=single
  Logical Operator : Logic  Operator=OR  AllPortsSameDT=off  OutDataTypeStr=boolean
  Switch2 : Switch  Criteria=u2 ~= 0  OutDataTypeStr=Inherit: Inherit via back propagation
  Switch3 : Switch  Criteria=u2 ~= 0  OutDataTypeStr=Inherit: Inherit via back propagation
  Switch8 : Switch  Criteria=u2 ~= 0  OutDataTypeStr=Inherit: Inherit via back propagation
  inv Lookup Table : Lookup_n-D  NumberOfTableDimensions=1  BreakpointsForDimension1=frac_lut_table_breaks_coarse_cfo  IndexSearchMethod=Evenly spaced points  Table=frac_lut_table_data_coarse_cfo  InterpMethod=Flat  DiagnosticForOutOfRangeInput=Error  RemoveProtectionInput=on  InternalRulePriority=Speed  OutDataTypeStr=Inherit: Inherit via back propagation  RndMeth=Simplest  InputSameDT=on
  mult_delay : Delay  DelayLength=cr_mult_pipeline*2
  mult_delay_match : Delay  DelayLength=cr_mult_pipeline*2
  mult_delay_match1 : Delay  DelayLength=cr_mult_pipeline*2
  pipeline_delay1 : Delay  DelayLength=regular_pipeline
  pipeline_delay2 : Delay  DelayLength=regular_pipeline  InitialCondition=1
  pipeline_delay_match : Delay  DelayLength=regular_pipeline*2
  pipeline_delay_match1 : Delay  DelayLength=regular_pipeline*2
  Out : Outport
  wires:
  pipeline_delay2/1 -> Data Type Duplicate2/1, Switch2/3
  mult_delay/1 -> inv Lookup Table/1
  pipeline_delay1/1 -> mult_delay/1
  mult_delay_match1/1 -> Switch3/2
  mult_delay_match/1 -> Switch2/2
  pipeline_delay_match1/1 -> mult_delay_match1/1
  pipeline_delay_match/1 -> mult_delay_match/1
  inv Lookup Table/1 -> Data Type Duplicate/2, pipeline_delay2/1
  Switch8/1 -> Data Type Conversion/1
  Constant11/1 -> Switch8/1
  Logical Operator/1 -> Switch8/2
  Switch3/1 -> Data Type Duplicate2/2, Data Type Duplicate1/2, Out/1
  Constant4/1 -> Switch3/1
  Switch2/1 -> Data Type Duplicate1/1, Switch3/3
  Constant3/1 -> Switch2/1
  Compare To Constant4/1 -> pipeline_delay_match1/1, Logical Operator/2
  Compare To Constant1/1 -> pipeline_delay_match/1, Logical Operator/1
  In/1 -> Data Type Duplicate/1, Compare To Constant4/1, Compare To Constant1/1, Switch8/3
  Data Type Conversion/1 -> pipeline_delay1/1
